simulink model "SecRwRtStLtwdRtwdCtrl"  (R2018b)
settings: Solver=FixedStepDiscrete  StartTime=0.0  StopTime=10.0  FixedStep=0.01  RelTol=1e-3
undefined symbols (not defined in the file or in its folder): KeSMSuMdMotFinshdTm_Val, KeSMSuMdRetryTm1_Val, KeSMSuModeReqDurgTm_Val, KeSMSwSecRwRtStLtwdRtwdEnTrigBitMask_Val
libraries: StCtrlLib x1
settings Model: Creator=sn2xws  LastModifiedBy=sn2xws
settings DataIOCC: SaveFormat=StructureWithTime
settings OptimizationCC: DefaultParameterBehavior=Inlined  EnhancedBackFolding=on  PassReuseOutputArgsAs=Individual arguments  ZeroExternalMemoryAtStartup=off  ZeroInternalMemoryAtStartup=off  OptimizeBlockOrder=speed  DifferentSizesBufferReuse=on  OptimizationCustomize=off
settings DebuggingCC: ParameterTunabilityLossMsg=error
settings ModelReferenceCC: ModelReferenceNumInstancesAllowed=Single
settings SFSimCC: MATLABDynamicMemAlloc=off
settings RTWCC: SystemTargetFile=autosar.tlc  GenCodeOnly=on  TemplateMakefile=ert_default_tmf  Description=AUTOSAR  GenerateReport=on  IncludeHyperlinkInReport=on  LaunchReport=on  GenerateTraceInfo=on  GenerateTraceReport=on  GenerateTraceReportSl=on  GenerateTraceReportSf=on  GenerateTraceReportEml=on
settings CodeAppCC: ForceParamTrailComments=on  IgnoreCustomStorageClasses=off  OperatorAnnotations=on  SimulinkDataObjDesc=on  SFDataObjDesc=on  InsertBlockDesc=on
settings STFCustomTargetCC: TargetLangStandard=C99 (ISO)  MultiwordLength=256  ParMdlRefBuildCompliant=on  CompOptLevelCompliant=on  IncludeMdlTerminateFcn=off  CombineOutputUpdateFcns=on  SuppressErrorStatus=on  ERTCustomFileBanners=on  SupportNonFinite=off  SupportComplex=off  SupportContinuousTime=off  SupportNonInlinedSFcns=off  RemoveResetFunc=on  MATLABClassNameForMDSCustomization=Simulink.SoftwareTarget.ERTCustomization  AutosarCompliant=on  UseToolchainInfoCompliant=on  LookupTableObjectStructAxisOrder=2,1,3,4,...  LUTObjectStructOrderEvenSpacing=Size,Table,Breakpoints  SystemTargetFile=autosar.tlc
settings ERTTargetCC: TargetLangStandard=C99 (ISO)  ConcurrentExecutionCompliant=off  IncludeMdlTerminateFcn=off  SuppressErrorStatus=on  SupportNonFinite=off  SupportComplex=off  ModelStepFunctionPrototypeControlCompliant=off  CPPClassGenCompliant=off  AutosarCompliant=on  LookupTableObjectStructAxisOrder=2,1,3,4,...  LUTObjectStructOrderEvenSpacing=Size,Table,Breakpoints  InlinedParameterPlacement=NonHierarchical  ERTCustomFileTemplate=example_file_process.tlc  ERTFilePackagingFormat=Compact

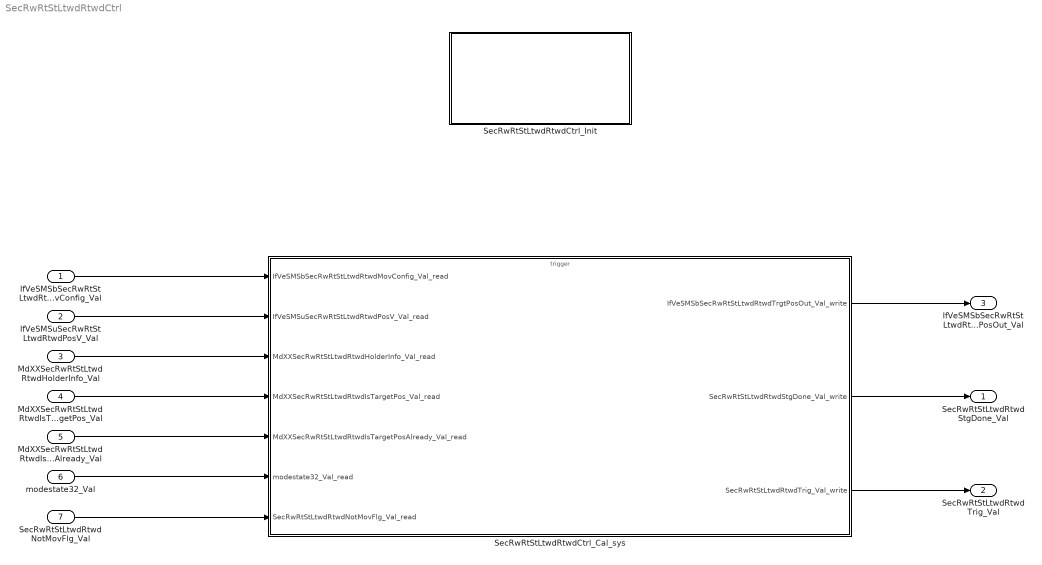
== system SecRwRtStLtwdRtwdCtrl ==
  IfVeSMSbSecRwRtStLtwdRtwdMovConfig_Val : Inport  OutDataTypeStr=boolean  PortDimensions=1
  IfVeSMSuSecRwRtStLtwdRtwdPosV_Val : Inport  Port=2  OutDataTypeStr=boolean  PortDimensions=1
  MdXXSecRwRtStLtwdRtwdHolderInfo_Val : Inport  Port=3  OutDataTypeStr=uint32  PortDimensions=1
  MdXXSecRwRtStLtwdRtwdIsTargetPos_Val : Inport  Port=4  OutDataTypeStr=uint32  PortDimensions=1
  MdXXSecRwRtStLtwdRtwdIsTargetPosAlready_Val : Inport  Port=5  OutDataTypeStr=uint32  PortDimensions=1
  modestate32_Val : Inport  Port=6  OutDataTypeStr=uint32  PortDimensions=1
  SecRwRtStLtwdRtwdNotMovFlg_Val : Inport  Port=7  OutDataTypeStr=boolean  PortDimensions=1
  SecRwRtStLtwdRtwdCtrl_Cal_sys : Subsystem
  SecRwRtStLtwdRtwdCtrl_Init : Subsystem
  SecRwRtStLtwdRtwdStgDone_Val : Outport  OutDataTypeStr=boolean  PortDimensions=1
  SecRwRtStLtwdRtwdTrig_Val : Outport  Port=2  OutDataTypeStr=boolean  PortDimensions=1
  IfVeSMSbSecRwRtStLtwdRtwdTrgtPosOut_Val : Outport  Port=3  OutDataTypeStr=boolean  PortDimensions=1
  wires:
  IfVeSMSbSecRwRtStLtwdRtwdMovConfig_Val/1 -> SecRwRtStLtwdRtwdCtrl_Cal_sys/1(IfVeSMSbSecRwRtStLtwdRtwdMovConfig_Val_read)
  IfVeSMSuSecRwRtStLtwdRtwdPosV_Val/1 -> SecRwRtStLtwdRtwdCtrl_Cal_sys/2(IfVeSMSuSecRwRtStLtwdRtwdPosV_Val_read)
  MdXXSecRwRtStLtwdRtwdHolderInfo_Val/1 -> SecRwRtStLtwdRtwdCtrl_Cal_sys/3(MdXXSecRwRtStLtwdRtwdHolderInfo_Val_read)
  MdXXSecRwRtStLtwdRtwdIsTargetPos_Val/1 -> SecRwRtStLtwdRtwdCtrl_Cal_sys/4(MdXXSecRwRtStLtwdRtwdIsTargetPos_Val_read)
  MdXXSecRwRtStLtwdRtwdIsTargetPosAlready_Val/1 -> SecRwRtStLtwdRtwdCtrl_Cal_sys/5(MdXXSecRwRtStLtwdRtwdIsTargetPosAlready_Val_read)
  modestate32_Val/1 -> SecRwRtStLtwdRtwdCtrl_Cal_sys/6(modestate32_Val_read)
  SecRwRtStLtwdRtwdNotMovFlg_Val/1 -> SecRwRtStLtwdRtwdCtrl_Cal_sys/7(SecRwRtStLtwdRtwdNotMovFlg_Val_read)
  SecRwRtStLtwdRtwdCtrl_Cal_sys/1(IfVeSMSbSecRwRtStLtwdRtwdTrgtPosOut_Val_write) -> IfVeSMSbSecRwRtStLtwdRtwdTrgtPosOut_Val/1
  SecRwRtStLtwdRtwdCtrl_Cal_sys/2(SecRwRtStLtwdRtwdStgDone_Val_write) -> SecRwRtStLtwdRtwdStgDone_Val/1
  SecRwRtStLtwdRtwdCtrl_Cal_sys/3(SecRwRtStLtwdRtwdTrig_Val_write) -> SecRwRtStLtwdRtwdTrig_Val/1

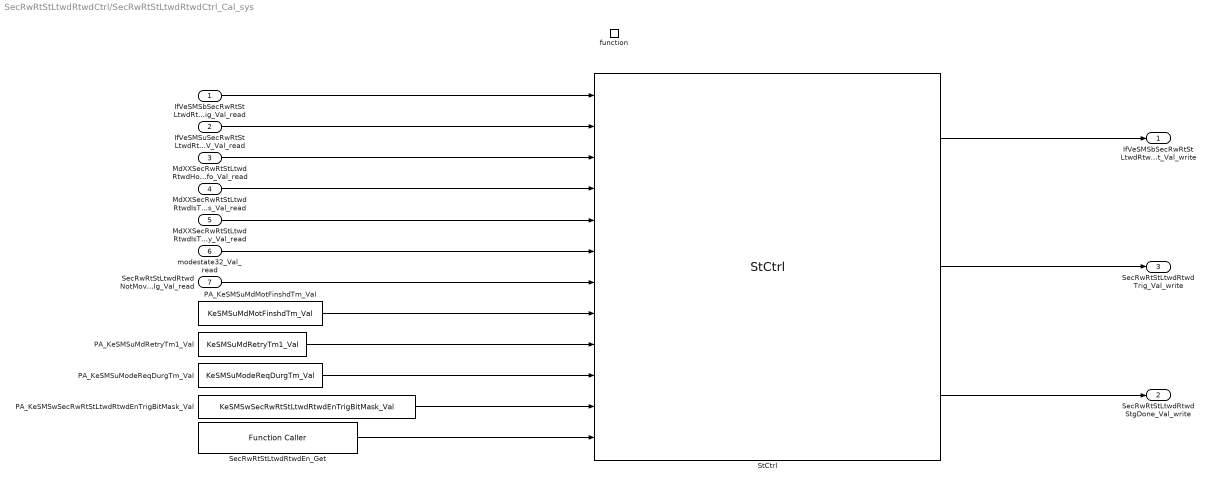
== system SecRwRtStLtwdRtwdCtrl/SecRwRtStLtwdRtwdCtrl_Cal_sys ==
  IfVeSMSbSecRwRtStLtwdRtwdMovConfig_Val_read : Inport
  IfVeSMSuSecRwRtStLtwdRtwdPosV_Val_read : Inport  Port=2
  MdXXSecRwRtStLtwdRtwdHolderInfo_Val_read : Inport  Port=3
  MdXXSecRwRtStLtwdRtwdIsTargetPos_Val_read : Inport  Port=4
  MdXXSecRwRtStLtwdRtwdIsTargetPosAlready_Val_read : Inport  Port=5
  modestate32_Val_read : Inport  Port=6
  SecRwRtStLtwdRtwdNotMovFlg_Val_read : Inport  Port=7
  function : TriggerPort  TriggerType=function-call  IsSimulinkFunction=on  FunctionName=SecRwRtStLtwdRtwdCtrl_Cal  VariantControl=(inherit)
  PA_KeSMSuMdMotFinshdTm_Val : Constant  Value=KeSMSuMdMotFinshdTm_Val
  PA_KeSMSuMdRetryTm1_Val : Constant  Value=KeSMSuMdRetryTm1_Val
  PA_KeSMSuModeReqDurgTm_Val : Constant  Value=KeSMSuModeReqDurgTm_Val
  PA_KeSMSwSecRwRtStLtwdRtwdEnTrigBitMask_Val : Constant  Value=KeSMSwSecRwRtStLtwdRtwdEnTrigBitMask_Val
  SecRwRtStLtwdRtwdEn_Get : FunctionCaller  FunctionPrototype=data = SecRwRtStLtwdRtwdEn_Get()  OutputArgumentSpecifications=uint32(1)
  StCtrl : StCtrlLib/StCtrl  SystemSampleTime=-1
  IfVeSMSbSecRwRtStLtwdRtwdTrgtPosOut_Val_write : Outport
      settings: EnsureOutportIsVirtual=on
  SecRwRtStLtwdRtwdStgDone_Val_write : Outport  Port=2
      settings: EnsureOutportIsVirtual=on
  SecRwRtStLtwdRtwdTrig_Val_write : Outport  Port=3
      settings: EnsureOutportIsVirtual=on
  wires:
  StCtrl/1 -> IfVeSMSbSecRwRtStLtwdRtwdTrgtPosOut_Val_write/1
  StCtrl/3 -> SecRwRtStLtwdRtwdStgDone_Val_write/1
  StCtrl/2 -> SecRwRtStLtwdRtwdTrig_Val_write/1
  PA_KeSMSwSecRwRtStLtwdRtwdEnTrigBitMask_Val/1 -> StCtrl/11
  SecRwRtStLtwdRtwdEn_Get/1 -> StCtrl/12
  PA_KeSMSuMdMotFinshdTm_Val/1 -> StCtrl/8
  PA_KeSMSuModeReqDurgTm_Val/1 -> StCtrl/10
  PA_KeSMSuMdRetryTm1_Val/1 -> StCtrl/9
  IfVeSMSbSecRwRtStLtwdRtwdMovConfig_Val_read/1 -> StCtrl/1
  IfVeSMSuSecRwRtStLtwdRtwdPosV_Val_read/1 -> StCtrl/2
  MdXXSecRwRtStLtwdRtwdHolderInfo_Val_read/1 -> StCtrl/3
  MdXXSecRwRtStLtwdRtwdIsTargetPos_Val_read/1 -> StCtrl/4
  MdXXSecRwRtStLtwdRtwdIsTargetPosAlready_Val_read/1 -> StCtrl/5
  modestate32_Val_read/1 -> StCtrl/6
  SecRwRtStLtwdRtwdNotMovFlg_Val_read/1 -> StCtrl/7

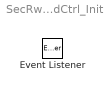
== system SecRwRtStLtwdRtwdCtrl/SecRwRtStLtwdRtwdCtrl_Init ==
  Event Listener : EventListener  EventName=reset
